simulink model "orion_casestudy_8"  (R2023a)
settings: Solver=VariableStepAuto  StartTime=0.0  StopTime=30  RelTol=1e-3
InitFcn:
  | RandStream.setGlobalStream(RandStream('mt19937ar','seed',sum(100*clock)));
undefined symbols (not defined in the file or in its folder): m, n
(part 1 of 3)
settings Model: Creator=simon  LastModifiedBy=simon
settings OptimizationCC: AccelVerboseBuild=on
settings DebuggingCC: UnderSpecifiedDataTypeMsg=warning  UnderSpecifiedDimensionMsg=warning

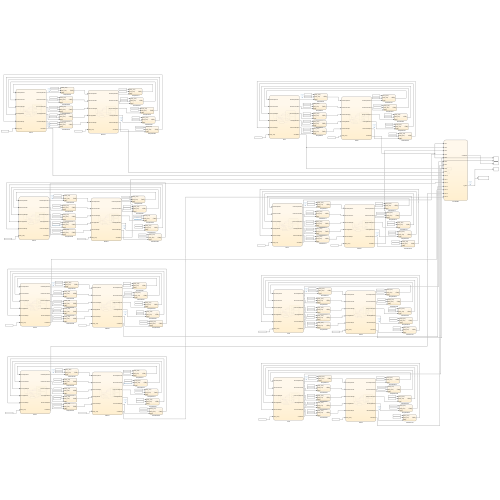
[thumbnail: Simulink's stored preview of the top-level diagram]
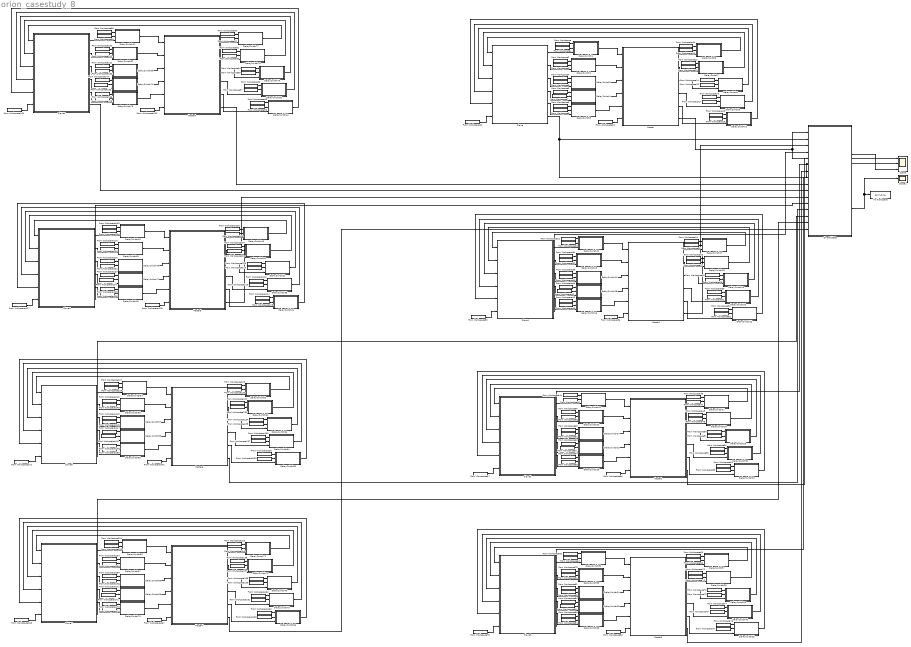
== system orion_casestudy_8 ==
  DelaySwitch1 : Stateflow chart  TreatAsAtomicUnit=on
  DelaySwitch10 : Stateflow chart  TreatAsAtomicUnit=on
  DelaySwitch11 : Stateflow chart  TreatAsAtomicUnit=on
  DelaySwitch12 : Stateflow chart  TreatAsAtomicUnit=on
  DelaySwitch13 : Stateflow chart  TreatAsAtomicUnit=on
  DelaySwitch14 : Stateflow chart  TreatAsAtomicUnit=on
  DelaySwitch15 : Stateflow chart  TreatAsAtomicUnit=on
  DelaySwitch16 : Stateflow chart  TreatAsAtomicUnit=on
  DelaySwitch17 : Stateflow chart  TreatAsAtomicUnit=on
  DelaySwitch18 : Stateflow chart  TreatAsAtomicUnit=on
  DelaySwitch19 : Stateflow chart  TreatAsAtomicUnit=on
  DelaySwitch2 : Stateflow chart  TreatAsAtomicUnit=on
  DelaySwitch20 : Stateflow chart  TreatAsAtomicUnit=on
  DelaySwitch21 : Stateflow chart  TreatAsAtomicUnit=on
  DelaySwitch22 : Stateflow chart  TreatAsAtomicUnit=on
  DelaySwitch23 : Stateflow chart  TreatAsAtomicUnit=on
  DelaySwitch24 : Stateflow chart  TreatAsAtomicUnit=on
  DelaySwitch25 : Stateflow chart  TreatAsAtomicUnit=on
  DelaySwitch26 : Stateflow chart  TreatAsAtomicUnit=on
  DelaySwitch27 : Stateflow chart  TreatAsAtomicUnit=on
  DelaySwitch28 : Stateflow chart  TreatAsAtomicUnit=on
  DelaySwitch29 : Stateflow chart  TreatAsAtomicUnit=on
  DelaySwitch3 : Stateflow chart  TreatAsAtomicUnit=on
  DelaySwitch30 : Stateflow chart  TreatAsAtomicUnit=on
  DelaySwitch31 : Stateflow chart  TreatAsAtomicUnit=on
  DelaySwitch32 : Stateflow chart  TreatAsAtomicUnit=on
  DelaySwitch33 : Stateflow chart  TreatAsAtomicUnit=on
  DelaySwitch34 : Stateflow chart  TreatAsAtomicUnit=on
  DelaySwitch35 : Stateflow chart  TreatAsAtomicUnit=on
  DelaySwitch36 : Stateflow chart  TreatAsAtomicUnit=on
  DelaySwitch37 : Stateflow chart  TreatAsAtomicUnit=on
  DelaySwitch38 : Stateflow chart  TreatAsAtomicUnit=on
  DelaySwitch39 : Stateflow chart  TreatAsAtomicUnit=on
  DelaySwitch4 : Stateflow chart  TreatAsAtomicUnit=on
  DelaySwitch40 : Stateflow chart  TreatAsAtomicUnit=on
  DelaySwitch41 : Stateflow chart  TreatAsAtomicUnit=on
  DelaySwitch42 : Stateflow chart  TreatAsAtomicUnit=on
  DelaySwitch43 : Stateflow chart  TreatAsAtomicUnit=on
  DelaySwitch44 : Stateflow chart  TreatAsAtomicUnit=on
  DelaySwitch45 : Stateflow chart  TreatAsAtomicUnit=on
  DelaySwitch46 : Stateflow chart  TreatAsAtomicUnit=on
  DelaySwitch47 : Stateflow chart  TreatAsAtomicUnit=on
  DelaySwitch48 : Stateflow chart  TreatAsAtomicUnit=on
  DelaySwitch49 : Stateflow chart  TreatAsAtomicUnit=on
  DelaySwitch5 : Stateflow chart  TreatAsAtomicUnit=on
  DelaySwitch50 : Stateflow chart  TreatAsAtomicUnit=on
  DelaySwitch51 : Stateflow chart  TreatAsAtomicUnit=on
  DelaySwitch52 : Stateflow chart  TreatAsAtomicUnit=on
  DelaySwitch53 : Stateflow chart  TreatAsAtomicUnit=on
  DelaySwitch54 : Stateflow chart  TreatAsAtomicUnit=on
  DelaySwitch55 : Stateflow chart  TreatAsAtomicUnit=on
  DelaySwitch56 : Stateflow chart  TreatAsAtomicUnit=on
  DelaySwitch57 : Stateflow chart  TreatAsAtomicUnit=on
  DelaySwitch58 : Stateflow chart  TreatAsAtomicUnit=on
  DelaySwitch59 : Stateflow chart  TreatAsAtomicUnit=on
  DelaySwitch6 : Stateflow chart  TreatAsAtomicUnit=on
  DelaySwitch60 : Stateflow chart  TreatAsAtomicUnit=on
  DelaySwitch61 : Stateflow chart  TreatAsAtomicUnit=on
  DelaySwitch62 : Stateflow chart  TreatAsAtomicUnit=on
  DelaySwitch63 : Stateflow chart  TreatAsAtomicUnit=on
  DelaySwitch64 : Stateflow chart  TreatAsAtomicUnit=on
  DelaySwitch65 : Stateflow chart  TreatAsAtomicUnit=on
  DelaySwitch66 : Stateflow chart  TreatAsAtomicUnit=on
  DelaySwitch67 : Stateflow chart  TreatAsAtomicUnit=on
  DelaySwitch68 : Stateflow chart  TreatAsAtomicUnit=on
  DelaySwitch69 : Stateflow chart  TreatAsAtomicUnit=on
  DelaySwitch7 : Stateflow chart  TreatAsAtomicUnit=on
  DelaySwitch70 : Stateflow chart  TreatAsAtomicUnit=on
  DelaySwitch71 : Stateflow chart  TreatAsAtomicUnit=on
  DelaySwitch72 : Stateflow chart  TreatAsAtomicUnit=on
  DelaySwitch73 : Stateflow chart  TreatAsAtomicUnit=on
  DelaySwitch74 : Stateflow chart  TreatAsAtomicUnit=on
  DelaySwitch75 : Stateflow chart  TreatAsAtomicUnit=on
  DelaySwitch76 : Stateflow chart  TreatAsAtomicUnit=on
  DelaySwitch77 : Stateflow chart  TreatAsAtomicUnit=on
  DelaySwitch78 : Stateflow chart  TreatAsAtomicUnit=on
  DelaySwitch79 : Stateflow chart  TreatAsAtomicUnit=on
  DelaySwitch8 : Stateflow chart  TreatAsAtomicUnit=on
  DelaySwitch80 : Stateflow chart  TreatAsAtomicUnit=on
  DelaySwitch9 : Stateflow chart  TreatAsAtomicUnit=on
  From Workspace : FromWorkspace  VariableName=switch_array_1  SampleTime=-1  Interpolate=off  ZeroCross=off  OutputAfterFinalValue=Holding final value
  From Workspace1 : FromWorkspace  VariableName=delay_array_1  SampleTime=-1  Interpolate=off  ZeroCross=off  OutputAfterFinalValue=Holding final value
  From Workspace10 : FromWorkspace  VariableName=switch_array_6  SampleTime=-1  Interpolate=off  ZeroCross=off  OutputAfterFinalValue=Holding final value
  From Workspace100 : FromWorkspace  VariableName=switch_array_52  SampleTime=-1  Interpolate=off  ZeroCross=off  OutputAfterFinalValue=Holding final value
  From Workspace101 : FromWorkspace  VariableName=delay_array_S5  SampleTime=-1  Interpolate=off  ZeroCross=off  OutputAfterFinalValue=Holding final value
  From Workspace102 : FromWorkspace  VariableName=delay_array_M5  SampleTime=-1  Interpolate=off  ZeroCross=off  OutputAfterFinalValue=Holding final value
  From Workspace103 : FromWorkspace  VariableName=switch_array_61  SampleTime=-1  Interpolate=off  ZeroCross=off  OutputAfterFinalValue=Holding final value
  From Workspace104 : FromWorkspace  VariableName=delay_array_61  SampleTime=-1  Interpolate=off  ZeroCross=off  OutputAfterFinalValue=Holding final value
  From Workspace105 : FromWorkspace  VariableName=switch_array_66  SampleTime=-1  Interpolate=off  ZeroCross=off  OutputAfterFinalValue=Holding final value
  From Workspace106 : FromWorkspace  VariableName=delay_array_66  SampleTime=-1  Interpolate=off  ZeroCross=off  OutputAfterFinalValue=Holding final value
  From Workspace107 : FromWorkspace  VariableName=switch_array_67  SampleTime=-1  Interpolate=off  ZeroCross=off  OutputAfterFinalValue=Holding final value
  From Workspace108 : FromWorkspace  VariableName=delay_array_67  SampleTime=-1  Interpolate=off  ZeroCross=off  OutputAfterFinalValue=Holding final value
  From Workspace109 : FromWorkspace  VariableName=switch_array_68  SampleTime=-1  Interpolate=off  ZeroCross=off  OutputAfterFinalValue=Holding final value
  From Workspace11 : FromWorkspace  VariableName=delay_array_6  SampleTime=-1  Interpolate=off  ZeroCross=off  OutputAfterFinalValue=Holding final value
  From Workspace110 : FromWorkspace  VariableName=delay_array_68  SampleTime=-1  Interpolate=off  ZeroCross=off  OutputAfterFinalValue=Holding final value
  From Workspace111 : FromWorkspace  VariableName=delay_array_52  SampleTime=-1  Interpolate=off  ZeroCross=off  OutputAfterFinalValue=Holding final value
  From Workspace112 : FromWorkspace  VariableName=switch_array_69  SampleTime=-1  Interpolate=off  ZeroCross=off  OutputAfterFinalValue=Holding final value
  From Workspace113 : FromWorkspace  VariableName=delay_array_69  SampleTime=-1  Interpolate=off  ZeroCross=off  OutputAfterFinalValue=Holding final value
  From Workspace114 : FromWorkspace  VariableName=switch_array_70  SampleTime=-1  Interpolate=off  ZeroCross=off  OutputAfterFinalValue=Holding final value
  From Workspace115 : FromWorkspace  VariableName=delay_array_70  SampleTime=-1  Interpolate=off  ZeroCross=off  OutputAfterFinalValue=Holding final value
  From Workspace116 : FromWorkspace  VariableName=switch_array_62  SampleTime=-1  Interpolate=off  ZeroCross=off  OutputAfterFinalValue=Holding final value
  From Workspace117 : FromWorkspace  VariableName=delay_array_S6  SampleTime=-1  Interpolate=off  ZeroCross=off  OutputAfterFinalValue=Holding final value
  From Workspace118 : FromWorkspace  VariableName=delay_array_M6  SampleTime=-1  Interpolate=off  ZeroCross=off  OutputAfterFinalValue=Holding final value
  From Workspace119 : FromWorkspace  VariableName=delay_array_62  SampleTime=-1  Interpolate=off  ZeroCross=off  OutputAfterFinalValue=Holding final value
  From Workspace12 : FromWorkspace  VariableName=switch_array_7  SampleTime=-1  Interpolate=off  ZeroCross=off  OutputAfterFinalValue=Holding final value
  From Workspace120 : FromWorkspace  VariableName=switch_array_63  SampleTime=-1  Interpolate=off  ZeroCross=off  OutputAfterFinalValue=Holding final value
  From Workspace121 : FromWorkspace  VariableName=delay_array_63  SampleTime=-1  Interpolate=off  ZeroCross=off  OutputAfterFinalValue=Holding final value
  From Workspace122 : FromWorkspace  VariableName=switch_array_53  SampleTime=-1  Interpolate=off  ZeroCross=off  OutputAfterFinalValue=Holding final value
  From Workspace123 : FromWorkspace  VariableName=switch_array_64  SampleTime=-1  Interpolate=off  ZeroCross=off  OutputAfterFinalValue=Holding final value
  From Workspace124 : FromWorkspace  VariableName=delay_array_64  SampleTime=-1  Interpolate=off  ZeroCross=off  OutputAfterFinalValue=Holding final value
  From Workspace125 : FromWorkspace  VariableName=switch_array_65  SampleTime=-1  Interpolate=off  ZeroCross=off  OutputAfterFinalValue=Holding final value
  From Workspace126 : FromWorkspace  VariableName=delay_array_65  SampleTime=-1  Interpolate=off  ZeroCross=off  OutputAfterFinalValue=Holding final value
  From Workspace127 : FromWorkspace  VariableName=switch_array_71  SampleTime=-1  Interpolate=off  ZeroCross=off  OutputAfterFinalValue=Holding final value
  From Workspace128 : FromWorkspace  VariableName=delay_array_71  SampleTime=-1  Interpolate=off  ZeroCross=off  OutputAfterFinalValue=Holding final value
  From Workspace129 : FromWorkspace  VariableName=switch_array_76  SampleTime=-1  Interpolate=off  ZeroCross=off  OutputAfterFinalValue=Holding final value
  From Workspace13 : FromWorkspace  VariableName=delay_array_7  SampleTime=-1  Interpolate=off  ZeroCross=off  OutputAfterFinalValue=Holding final value
  From Workspace130 : FromWorkspace  VariableName=delay_array_76  SampleTime=-1  Interpolate=off  ZeroCross=off  OutputAfterFinalValue=Holding final value
  From Workspace131 : FromWorkspace  VariableName=switch_array_77  SampleTime=-1  Interpolate=off  ZeroCross=off  OutputAfterFinalValue=Holding final value
  From Workspace132 : FromWorkspace  VariableName=delay_array_77  SampleTime=-1  Interpolate=off  ZeroCross=off  OutputAfterFinalValue=Holding final value
  From Workspace133 : FromWorkspace  VariableName=delay_array_53  SampleTime=-1  Interpolate=off  ZeroCross=off  OutputAfterFinalValue=Holding final value
  From Workspace134 : FromWorkspace  VariableName=switch_array_78  SampleTime=-1  Interpolate=off  ZeroCross=off  OutputAfterFinalValue=Holding final value
  From Workspace135 : FromWorkspace  VariableName=delay_array_78  SampleTime=-1  Interpolate=off  ZeroCross=off  OutputAfterFinalValue=Holding final value
  From Workspace136 : FromWorkspace  VariableName=switch_array_79  SampleTime=-1  Interpolate=off  ZeroCross=off  OutputAfterFinalValue=Holding final value
  From Workspace137 : FromWorkspace  VariableName=delay_array_79  SampleTime=-1  Interpolate=off  ZeroCross=off  OutputAfterFinalValue=Holding final value
  From Workspace138 : FromWorkspace  VariableName=switch_array_80  SampleTime=-1  Interpolate=off  ZeroCross=off  OutputAfterFinalValue=Holding final value
  From Workspace139 : FromWorkspace  VariableName=delay_array_80  SampleTime=-1  Interpolate=off  ZeroCross=off  OutputAfterFinalValue=Holding final value
  From Workspace14 : FromWorkspace  VariableName=switch_array_8  SampleTime=-1  Interpolate=off  ZeroCross=off  OutputAfterFinalValue=Holding final value
  From Workspace140 : FromWorkspace  VariableName=switch_array_72  SampleTime=-1  Interpolate=off  ZeroCross=off  OutputAfterFinalValue=Holding final value
  From Workspace141 : FromWorkspace  VariableName=delay_array_S7  SampleTime=-1  Interpolate=off  ZeroCross=off  OutputAfterFinalValue=Holding final value
  From Workspace142 : FromWorkspace  VariableName=delay_array_M7  SampleTime=-1  Interpolate=off  ZeroCross=off  OutputAfterFinalValue=Holding final value
  From Workspace143 : FromWorkspace  VariableName=delay_array_72  SampleTime=-1  Interpolate=off  ZeroCross=off  OutputAfterFinalValue=Holding final value
  From Workspace144 : FromWorkspace  VariableName=switch_array_54  SampleTime=-1  Interpolate=off  ZeroCross=off  OutputAfterFinalValue=Holding final value
  From Workspace145 : FromWorkspace  VariableName=switch_array_73  SampleTime=-1  Interpolate=off  ZeroCross=off  OutputAfterFinalValue=Holding final value
  From Workspace146 : FromWorkspace  VariableName=delay_array_73  SampleTime=-1  Interpolate=off  ZeroCross=off  OutputAfterFinalValue=Holding final value
  From Workspace147 : FromWorkspace  VariableName=switch_array_74  SampleTime=-1  Interpolate=off  ZeroCross=off  OutputAfterFinalValue=Holding final value
  From Workspace148 : FromWorkspace  VariableName=delay_array_74  SampleTime=-1  Interpolate=off  ZeroCross=off  OutputAfterFinalValue=Holding final value
  From Workspace149 : FromWorkspace  VariableName=switch_array_75  SampleTime=-1  Interpolate=off  ZeroCross=off  OutputAfterFinalValue=Holding final value
  From Workspace15 : FromWorkspace  VariableName=delay_array_8  SampleTime=-1  Interpolate=off  ZeroCross=off  OutputAfterFinalValue=Holding final value
  From Workspace150 : FromWorkspace  VariableName=delay_array_75  SampleTime=-1  Interpolate=off  ZeroCross=off  OutputAfterFinalValue=Holding final value
  From Workspace151 : FromWorkspace  VariableName=switch_array_81  SampleTime=-1  Interpolate=off  ZeroCross=off  OutputAfterFinalValue=Holding final value
  From Workspace152 : FromWorkspace  VariableName=delay_array_81  SampleTime=-1  Interpolate=off  ZeroCross=off  OutputAfterFinalValue=Holding final value
  From Workspace153 : FromWorkspace  VariableName=switch_array_86  SampleTime=-1  Interpolate=off  ZeroCross=off  OutputAfterFinalValue=Holding final value
  From Workspace154 : FromWorkspace  VariableName=delay_array_86  SampleTime=-1  Interpolate=off  ZeroCross=off  OutputAfterFinalValue=Holding final value
  From Workspace155 : FromWorkspace  VariableName=delay_array_54  SampleTime=-1  Interpolate=off  ZeroCross=off  OutputAfterFinalValue=Holding final value
  From Workspace156 : FromWorkspace  VariableName=switch_array_87  SampleTime=-1  Interpolate=off  ZeroCross=off  OutputAfterFinalValue=Holding final value
  From Workspace157 : FromWorkspace  VariableName=delay_array_87  SampleTime=-1  Interpolate=off  ZeroCross=off  OutputAfterFinalValue=Holding final value
  From Workspace158 : FromWorkspace  VariableName=switch_array_88  SampleTime=-1  Interpolate=off  ZeroCross=off  OutputAfterFinalValue=Holding final value
  From Workspace159 : FromWorkspace  VariableName=delay_array_88  SampleTime=-1  Interpolate=off  ZeroCross=off  OutputAfterFinalValue=Holding final value
  From Workspace16 : FromWorkspace  VariableName=switch_array_9  SampleTime=-1  Interpolate=off  ZeroCross=off  OutputAfterFinalValue=Holding final value
  From Workspace160 : FromWorkspace  VariableName=switch_array_89  SampleTime=-1  Interpolate=off  ZeroCross=off  OutputAfterFinalValue=Holding final value
  From Workspace161 : FromWorkspace  VariableName=delay_array_89  SampleTime=-1  Interpolate=off  ZeroCross=off  OutputAfterFinalValue=Holding final value
  From Workspace162 : FromWorkspace  VariableName=switch_array_90  SampleTime=-1  Interpolate=off  ZeroCross=off  OutputAfterFinalValue=Holding final value
  From Workspace163 : FromWorkspace  VariableName=delay_array_90  SampleTime=-1  Interpolate=off  ZeroCross=off  OutputAfterFinalValue=Holding final value
  From Workspace164 : FromWorkspace  VariableName=switch_array_82  SampleTime=-1  Interpolate=off  ZeroCross=off  OutputAfterFinalValue=Holding final value
  From Workspace165 : FromWorkspace  VariableName=delay_array_S8  SampleTime=-1  Interpolate=off  ZeroCross=off  OutputAfterFinalValue=Holding final value
  From Workspace166 : FromWorkspace  VariableName=switch_array_55  SampleTime=-1  Interpolate=off  ZeroCross=off  OutputAfterFinalValue=Holding final value
  From Workspace167 : FromWorkspace  VariableName=delay_array_M8  SampleTime=-1  Interpolate=off  ZeroCross=off  OutputAfterFinalValue=Holding final value
  From Workspace168 : FromWorkspace  VariableName=delay_array_82  SampleTime=-1  Interpolate=off  ZeroCross=off  OutputAfterFinalValue=Holding final value
  From Workspace169 : FromWorkspace  VariableName=switch_array_83  SampleTime=-1  Interpolate=off  ZeroCross=off  OutputAfterFinalValue=Holding final value
  From Workspace17 : FromWorkspace  VariableName=delay_array_9  SampleTime=-1  Interpolate=off  ZeroCross=off  OutputAfterFinalValue=Holding final value
  From Workspace170 : FromWorkspace  VariableName=delay_array_83  SampleTime=-1  Interpolate=off  ZeroCross=off  OutputAfterFinalValue=Holding final value
  From Workspace171 : FromWorkspace  VariableName=switch_array_84  SampleTime=-1  Interpolate=off  ZeroCross=off  OutputAfterFinalValue=Holding final value
  From Workspace172 : FromWorkspace  VariableName=delay_array_84  SampleTime=-1  Interpolate=off  ZeroCross=off  OutputAfterFinalValue=Holding final value
  From Workspace173 : FromWorkspace  VariableName=switch_array_85  SampleTime=-1  Interpolate=off  ZeroCross=off  OutputAfterFinalValue=Holding final value
  From Workspace174 : FromWorkspace  VariableName=delay_array_85  SampleTime=-1  Interpolate=off  ZeroCross=off  OutputAfterFinalValue=Holding final value
  From Workspace175 : FromWorkspace  VariableName=delay_array_55  SampleTime=-1  Interpolate=off  ZeroCross=off  OutputAfterFinalValue=Holding final value
  From Workspace18 : FromWorkspace  VariableName=switch_array_10  SampleTime=-1  Interpolate=off  ZeroCross=off  OutputAfterFinalValue=Holding final value
  From Workspace19 : FromWorkspace  VariableName=delay_array_10  SampleTime=-1  Interpolate=off  ZeroCross=off  OutputAfterFinalValue=Holding final value
  From Workspace2 : FromWorkspace  VariableName=switch_array_2  SampleTime=-1  Interpolate=off  ZeroCross=off  OutputAfterFinalValue=Holding final value
  From Workspace20 : FromWorkspace  VariableName=delay_array_S1  SampleTime=-1  Interpolate=off  ZeroCross=off  OutputAfterFinalValue=Holding final value
  From Workspace21 : FromWorkspace  VariableName=delay_array_M1  SampleTime=-1  Interpolate=off  ZeroCross=off  OutputAfterFinalValue=Holding final value
  From Workspace22 : FromWorkspace  VariableName=switch_array_11  SampleTime=-1  Interpolate=off  ZeroCross=off  OutputAfterFinalValue=Holding final value
  From Workspace23 : FromWorkspace  VariableName=delay_array_11  SampleTime=-1  Interpolate=off  ZeroCross=off  OutputAfterFinalValue=Holding final value
  From Workspace24 : FromWorkspace  VariableName=switch_array_16  SampleTime=-1  Interpolate=off  ZeroCross=off  OutputAfterFinalValue=Holding final value
  From Workspace25 : FromWorkspace  VariableName=delay_array_16  SampleTime=-1  Interpolate=off  ZeroCross=off  OutputAfterFinalValue=Holding final value
  From Workspace26 : FromWorkspace  VariableName=switch_array_17  SampleTime=-1  Interpolate=off  ZeroCross=off  OutputAfterFinalValue=Holding final value
  From Workspace27 : FromWorkspace  VariableName=delay_array_17  SampleTime=-1  Interpolate=off  ZeroCross=off  OutputAfterFinalValue=Holding final value
  From Workspace28 : FromWorkspace  VariableName=switch_array_18  SampleTime=-1  Interpolate=off  ZeroCross=off  OutputAfterFinalValue=Holding final value
  From Workspace29 : FromWorkspace  VariableName=delay_array_18  SampleTime=-1  Interpolate=off  ZeroCross=off  OutputAfterFinalValue=Holding final value
  From Workspace3 : FromWorkspace  VariableName=delay_array_2  SampleTime=-1  Interpolate=off  ZeroCross=off  OutputAfterFinalValue=Holding final value
  From Workspace30 : FromWorkspace  VariableName=switch_array_19  SampleTime=-1  Interpolate=off  ZeroCross=off  OutputAfterFinalValue=Holding final value
  From Workspace31 : FromWorkspace  VariableName=delay_array_19  SampleTime=-1  Interpolate=off  ZeroCross=off  OutputAfterFinalValue=Holding final value
  From Workspace32 : FromWorkspace  VariableName=switch_array_20  SampleTime=-1  Interpolate=off  ZeroCross=off  OutputAfterFinalValue=Holding final value
  From Workspace33 : FromWorkspace  VariableName=delay_array_20  SampleTime=-1  Interpolate=off  ZeroCross=off  OutputAfterFinalValue=Holding final value
  From Workspace34 : FromWorkspace  VariableName=switch_array_12  SampleTime=-1  Interpolate=off  ZeroCross=off  OutputAfterFinalValue=Holding final value
  From Workspace35 : FromWorkspace  VariableName=delay_array_S2  SampleTime=-1  Interpolate=off  ZeroCross=off  OutputAfterFinalValue=Holding final value
  From Workspace36 : FromWorkspace  VariableName=delay_array_M2  SampleTime=-1  Interpolate=off  ZeroCross=off  OutputAfterFinalValue=Holding final value
  From Workspace37 : FromWorkspace  VariableName=delay_array_12  SampleTime=-1  Interpolate=off  ZeroCross=off  OutputAfterFinalValue=Holding final value
  From Workspace38 : FromWorkspace  VariableName=switch_array_13  SampleTime=-1  Interpolate=off  ZeroCross=off  OutputAfterFinalValue=Holding final value
  From Workspace39 : FromWorkspace  VariableName=delay_array_13  SampleTime=-1  Interpolate=off  ZeroCross=off  OutputAfterFinalValue=Holding final value
  From Workspace4 : FromWorkspace  VariableName=switch_array_3  SampleTime=-1  Interpolate=off  ZeroCross=off  OutputAfterFinalValue=Holding final value
  From Workspace40 : FromWorkspace  VariableName=switch_array_14  SampleTime=-1  Interpolate=off  ZeroCross=off  OutputAfterFinalValue=Holding final value
  From Workspace41 : FromWorkspace  VariableName=delay_array_14  SampleTime=-1  Interpolate=off  ZeroCross=off  OutputAfterFinalValue=Holding final value
  From Workspace42 : FromWorkspace  VariableName=switch_array_15  SampleTime=-1  Interpolate=off  ZeroCross=off  OutputAfterFinalValue=Holding final value
  From Workspace43 : FromWorkspace  VariableName=delay_array_15  SampleTime=-1  Interpolate=off  ZeroCross=off  OutputAfterFinalValue=Holding final value
  From Workspace44 : FromWorkspace  VariableName=switch_array_31  SampleTime=-1  Interpolate=off  ZeroCross=off  OutputAfterFinalValue=Holding final value
  From Workspace45 : FromWorkspace  VariableName=delay_array_31  SampleTime=-1  Interpolate=off  ZeroCross=off  OutputAfterFinalValue=Holding final value
  From Workspace46 : FromWorkspace  VariableName=switch_array_36  SampleTime=-1  Interpolate=off  ZeroCross=off  OutputAfterFinalValue=Holding final value
  From Workspace47 : FromWorkspace  VariableName=delay_array_36  SampleTime=-1  Interpolate=off  ZeroCross=off  OutputAfterFinalValue=Holding final value
  From Workspace48 : FromWorkspace  VariableName=switch_array_37  SampleTime=-1  Interpolate=off  ZeroCross=off  OutputAfterFinalValue=Holding final value
  From Workspace49 : FromWorkspace  VariableName=delay_array_37  SampleTime=-1  Interpolate=off  ZeroCross=off  OutputAfterFinalValue=Holding final value
  From Workspace5 : FromWorkspace  VariableName=delay_array_3  SampleTime=-1  Interpolate=off  ZeroCross=off  OutputAfterFinalValue=Holding final value
  From Workspace50 : FromWorkspace  VariableName=switch_array_38  SampleTime=-1  Interpolate=off  ZeroCross=off  OutputAfterFinalValue=Holding final value
  From Workspace51 : FromWorkspace  VariableName=delay_array_38  SampleTime=-1  Interpolate=off  ZeroCross=off  OutputAfterFinalValue=Holding final value
  From Workspace52 : FromWorkspace  VariableName=switch_array_39  SampleTime=-1  Interpolate=off  ZeroCross=off  OutputAfterFinalValue=Holding final value
  From Workspace53 : FromWorkspace  VariableName=delay_array_39  SampleTime=-1  Interpolate=off  ZeroCross=off  OutputAfterFinalValue=Holding final value
  From Workspace54 : FromWorkspace  VariableName=switch_array_40  SampleTime=-1  Interpolate=off  ZeroCross=off  OutputAfterFinalValue=Holding final value
  From Workspace55 : FromWorkspace  VariableName=delay_array_40  SampleTime=-1  Interpolate=off  ZeroCross=off  OutputAfterFinalValue=Holding final value
  From Workspace56 : FromWorkspace  VariableName=switch_array_32  SampleTime=-1  Interpolate=off  ZeroCross=off  OutputAfterFinalValue=Holding final value
  From Workspace57 : FromWorkspace  VariableName=delay_array_S3  SampleTime=-1  Interpolate=off  ZeroCross=off  OutputAfterFinalValue=Holding final value
  From Workspace58 : FromWorkspace  VariableName=delay_array_M3  SampleTime=-1  Interpolate=off  ZeroCross=off  OutputAfterFinalValue=Holding final value
  From Workspace59 : FromWorkspace  VariableName=delay_array_32  SampleTime=-1  Interpolate=off  ZeroCross=off  OutputAfterFinalValue=Holding final value
  From Workspace6 : FromWorkspace  VariableName=switch_array_4  SampleTime=-1  Interpolate=off  ZeroCross=off  OutputAfterFinalValue=Holding final value
  From Workspace60 : FromWorkspace  VariableName=switch_array_33  SampleTime=-1  Interpolate=off  ZeroCross=off  OutputAfterFinalValue=Holding final value
  From Workspace61 : FromWorkspace  VariableName=delay_array_33  SampleTime=-1  Interpolate=off  ZeroCross=off  OutputAfterFinalValue=Holding final value
  From Workspace62 : FromWorkspace  VariableName=switch_array_34  SampleTime=-1  Interpolate=off  ZeroCross=off  OutputAfterFinalValue=Holding final value
  From Workspace63 : FromWorkspace  VariableName=delay_array_34  SampleTime=-1  Interpolate=off  ZeroCross=off  OutputAfterFinalValue=Holding final value
  From Workspace64 : FromWorkspace  VariableName=switch_array_35  SampleTime=-1  Interpolate=off  ZeroCross=off  OutputAfterFinalValue=Holding final value
  From Workspace65 : FromWorkspace  VariableName=delay_array_35  SampleTime=-1  Interpolate=off  ZeroCross=off  OutputAfterFinalValue=Holding final value
  From Workspace66 : FromWorkspace  VariableName=switch_array_41  SampleTime=-1  Interpolate=off  ZeroCross=off  OutputAfterFinalValue=Holding final value
  From Workspace67 : FromWorkspace  VariableName=delay_array_41  SampleTime=-1  Interpolate=off  ZeroCross=off  OutputAfterFinalValue=Holding final value
  From Workspace68 : FromWorkspace  VariableName=switch_array_46  SampleTime=-1  Interpolate=off  ZeroCross=off  OutputAfterFinalValue=Holding final value
  From Workspace69 : FromWorkspace  VariableName=delay_array_46  SampleTime=-1  Interpolate=off  ZeroCross=off  OutputAfterFinalValue=Holding final value
  From Workspace7 : FromWorkspace  VariableName=delay_array_4  SampleTime=-1  Interpolate=off  ZeroCross=off  OutputAfterFinalValue=Holding final value
  From Workspace70 : FromWorkspace  VariableName=switch_array_47  SampleTime=-1  Interpolate=off  ZeroCross=off  OutputAfterFinalValue=Holding final value
  From Workspace71 : FromWorkspace  VariableName=delay_array_47  SampleTime=-1  Interpolate=off  ZeroCross=off  OutputAfterFinalValue=Holding final value
  From Workspace72 : FromWorkspace  VariableName=switch_array_48  SampleTime=-1  Interpolate=off  ZeroCross=off  OutputAfterFinalValue=Holding final value
  From Workspace73 : FromWorkspace  VariableName=delay_array_48  SampleTime=-1  Interpolate=off  ZeroCross=off  OutputAfterFinalValue=Holding final value
  From Workspace74 : FromWorkspace  VariableName=switch_array_49  SampleTime=-1  Interpolate=off  ZeroCross=off  OutputAfterFinalValue=Holding final value
  From Workspace75 : FromWorkspace  VariableName=delay_array_49  SampleTime=-1  Interpolate=off  ZeroCross=off  OutputAfterFinalValue=Holding final value
  From Workspace76 : FromWorkspace  VariableName=switch_array_50  SampleTime=-1  Interpolate=off  ZeroCross=off  OutputAfterFinalValue=Holding final value
  From Workspace77 : FromWorkspace  VariableName=delay_array_50  SampleTime=-1  Interpolate=off  ZeroCross=off  OutputAfterFinalValue=Holding final value
  From Workspace78 : FromWorkspace  VariableName=switch_array_42  SampleTime=-1  Interpolate=off  ZeroCross=off  OutputAfterFinalValue=Holding final value
  From Workspace79 : FromWorkspace  VariableName=delay_array_S4  SampleTime=-1  Interpolate=off  ZeroCross=off  OutputAfterFinalValue=Holding final value
  From Workspace8 : FromWorkspace  VariableName=switch_array_5  SampleTime=-1  Interpolate=off  ZeroCross=off  OutputAfterFinalValue=Holding final value
  From Workspace80 : FromWorkspace  VariableName=delay_array_M4  SampleTime=-1  Interpolate=off  ZeroCross=off  OutputAfterFinalValue=Holding final value
  From Workspace81 : FromWorkspace  VariableName=delay_array_42  SampleTime=-1  Interpolate=off  ZeroCross=off  OutputAfterFinalValue=Holding final value
  From Workspace82 : FromWorkspace  VariableName=switch_array_43  SampleTime=-1  Interpolate=off  ZeroCross=off  OutputAfterFinalValue=Holding final value
  From Workspace83 : FromWorkspace  VariableName=delay_array_43  SampleTime=-1  Interpolate=off  ZeroCross=off  OutputAfterFinalValue=Holding final value
  From Workspace84 : FromWorkspace  VariableName=switch_array_44  SampleTime=-1  Interpolate=off  ZeroCross=off  OutputAfterFinalValue=Holding final value
  From Workspace85 : FromWorkspace  VariableName=delay_array_44  SampleTime=-1  Interpolate=off  ZeroCross=off  OutputAfterFinalValue=Holding final value
  From Workspace86 : FromWorkspace  VariableName=switch_array_45  SampleTime=-1  Interpolate=off  ZeroCross=off  OutputAfterFinalValue=Holding final value
  From Workspace87 : FromWorkspace  VariableName=delay_array_45  SampleTime=-1  Interpolate=off  ZeroCross=off  OutputAfterFinalValue=Holding final value
  From Workspace88 : FromWorkspace  VariableName=switch_array_51  SampleTime=-1  Interpolate=off  ZeroCross=off  OutputAfterFinalValue=Holding final value
  From Workspace89 : FromWorkspace  VariableName=delay_array_51  SampleTime=-1  Interpolate=off  ZeroCross=off  OutputAfterFinalValue=Holding final value
  From Workspace9 : FromWorkspace  VariableName=delay_array_5  SampleTime=-1  Interpolate=off  ZeroCross=off  OutputAfterFinalValue=Holding final value
  From Workspace90 : FromWorkspace  VariableName=switch_array_56  SampleTime=-1  Interpolate=off  ZeroCross=off  OutputAfterFinalValue=Holding final value
  From Workspace91 : FromWorkspace  VariableName=delay_array_56  SampleTime=-1  Interpolate=off  ZeroCross=off  OutputAfterFinalValue=Holding final value
  From Workspace92 : FromWorkspace  VariableName=switch_array_57  SampleTime=-1  Interpolate=off  ZeroCross=off  OutputAfterFinalValue=Holding final value
  From Workspace93 : FromWorkspace  VariableName=delay_array_57  SampleTime=-1  Interpolate=off  ZeroCross=off  OutputAfterFinalValue=Holding final value
  From Workspace94 : FromWorkspace  VariableName=switch_array_58  SampleTime=-1  Interpolate=off  ZeroCross=off  OutputAfterFinalValue=Holding final value
  From Workspace95 : FromWorkspace  VariableName=delay_array_58  SampleTime=-1  Interpolate=off  ZeroCross=off  OutputAfterFinalValue=Holding final value
  From Workspace96 : FromWorkspace  VariableName=switch_array_59  SampleTime=-1  Interpolate=off  ZeroCross=off  OutputAfterFinalValue=Holding final value
  From Workspace97 : FromWorkspace  VariableName=delay_array_59  SampleTime=-1  Interpolate=off  ZeroCross=off  OutputAfterFinalValue=Holding final value
  From Workspace98 : FromWorkspace  VariableName=switch_array_60  SampleTime=-1  Interpolate=off  ZeroCross=off  OutputAfterFinalValue=Holding final value
  From Workspace99 : FromWorkspace  VariableName=delay_array_60  SampleTime=-1  Interpolate=off  ZeroCross=off  OutputAfterFinalValue=Holding final value
  Master : Stateflow chart  TreatAsAtomicUnit=on
      settings: PortSchema="{\"entries\":[{\"content\":{\"sides\":[{\"content\":{\"connectorIds\":[\"In2\",\"In3\",\"In5\",\"In4\",\"In6\",\"In1\"]},\"type\":\"ConnectorPlacement.EquallySpacedRectSide\",\"uuid\":\"93190a42-59cb-4d31-aa72-080cef5549db\"},{\"content\":{\"connectorIds\":[\"Out1\",\"Out2\",\"Out3\",\"Out4\",\"Out5\",\"Out6\"],\"side\":\"RIGHT\"},\"type\":\"ConnectorPlacement.EquallySpacedRectSide\",\"uuid\":\"4a04e977-42e8-4d3e-8e66-86884aeb71d4\"},{\"content\":{\"side\":\"TOP\"},\"type\":\"ConnectorPlacement.EquallySpacedRectSide\",\"uuid\":\"cb7bc3bf-3799-42a3-9f12-c8b4e7be85f7\"},{\"content\":{\"side\":\"BOTTOM\"},\"type\":\"ConnectorPlacement.EquallySpacedRectSide\",\"uuid\":\"934a78a5-af7b-46d0-ad43-c65a76addb63\"}]},\"type\":\"ConnectorPlacement.EquallySpacedConnector\",\"uuid\":\"bab253c4-7746-42e8-9b4d-6fa7ff1cc3b1\"}],\"packageUris\":[\"http://schema.mathworks.com/mf0/Connector/R2020b\"],\"version\":\"1.0\"}"
  Master1 : Stateflow chart  TreatAsAtomicUnit=on
      settings: PortSchema="{\"entries\":[{\"content\":{\"sides\":[{\"content\":{\"connectorIds\":[\"In2\",\"In3\",\"In5\",\"In4\",\"In6\",\"In1\"]},\"type\":\"ConnectorPlacement.EquallySpacedRectSide\",\"uuid\":\"93190a42-59cb-4d31-aa72-080cef5549db\"},{\"content\":{\"connectorIds\":[\"Out1\",\"Out2\",\"Out3\",\"Out4\",\"Out5\",\"Out6\"],\"side\":\"RIGHT\"},\"type\":\"ConnectorPlacement.EquallySpacedRectSide\",\"uuid\":\"4a04e977-42e8-4d3e-8e66-86884aeb71d4\"},{\"content\":{\"side\":\"TOP\"},\"type\":\"ConnectorPlacement.EquallySpacedRectSide\",\"uuid\":\"cb7bc3bf-3799-42a3-9f12-c8b4e7be85f7\"},{\"content\":{\"side\":\"BOTTOM\"},\"type\":\"ConnectorPlacement.EquallySpacedRectSide\",\"uuid\":\"934a78a5-af7b-46d0-ad43-c65a76addb63\"}]},\"type\":\"ConnectorPlacement.EquallySpacedConnector\",\"uuid\":\"bab253c4-7746-42e8-9b4d-6fa7ff1cc3b1\"}],\"packageUris\":[\"http://schema.mathworks.com/mf0/Connector/R2020b\"],\"version\":\"1.0\"}"
  Master2 : Stateflow chart  TreatAsAtomicUnit=on
      settings: PortSchema="{\"entries\":[{\"content\":{\"sides\":[{\"content\":{\"connectorIds\":[\"In2\",\"In3\",\"In5\",\"In4\",\"In6\",\"In1\"]},\"type\":\"ConnectorPlacement.EquallySpacedRectSide\",\"uuid\":\"93190a42-59cb-4d31-aa72-080cef5549db\"},{\"content\":{\"connectorIds\":[\"Out1\",\"Out2\",\"Out3\",\"Out4\",\"Out5\",\"Out6\"],\"side\":\"RIGHT\"},\"type\":\"ConnectorPlacement.EquallySpacedRectSide\",\"uuid\":\"4a04e977-42e8-4d3e-8e66-86884aeb71d4\"},{\"content\":{\"side\":\"TOP\"},\"type\":\"ConnectorPlacement.EquallySpacedRectSide\",\"uuid\":\"cb7bc3bf-3799-42a3-9f12-c8b4e7be85f7\"},{\"content\":{\"side\":\"BOTTOM\"},\"type\":\"ConnectorPlacement.EquallySpacedRectSide\",\"uuid\":\"934a78a5-af7b-46d0-ad43-c65a76addb63\"}]},\"type\":\"ConnectorPlacement.EquallySpacedConnector\",\"uuid\":\"bab253c4-7746-42e8-9b4d-6fa7ff1cc3b1\"}],\"packageUris\":[\"http://schema.mathworks.com/mf0/Connector/R2020b\"],\"version\":\"1.0\"}"
  Master3 : Stateflow chart  TreatAsAtomicUnit=on
      settings: PortSchema="{\"entries\":[{\"content\":{\"sides\":[{\"content\":{\"connectorIds\":[\"In2\",\"In3\",\"In5\",\"In4\",\"In6\",\"In1\"]},\"type\":\"ConnectorPlacement.EquallySpacedRectSide\",\"uuid\":\"93190a42-59cb-4d31-aa72-080cef5549db\"},{\"content\":{\"connectorIds\":[\"Out1\",\"Out2\",\"Out3\",\"Out4\",\"Out5\",\"Out6\"],\"side\":\"RIGHT\"},\"type\":\"ConnectorPlacement.EquallySpacedRectSide\",\"uuid\":\"4a04e977-42e8-4d3e-8e66-86884aeb71d4\"},{\"content\":{\"side\":\"TOP\"},\"type\":\"ConnectorPlacement.EquallySpacedRectSide\",\"uuid\":\"cb7bc3bf-3799-42a3-9f12-c8b4e7be85f7\"},{\"content\":{\"side\":\"BOTTOM\"},\"type\":\"ConnectorPlacement.EquallySpacedRectSide\",\"uuid\":\"934a78a5-af7b-46d0-ad43-c65a76addb63\"}]},\"type\":\"ConnectorPlacement.EquallySpacedConnector\",\"uuid\":\"bab253c4-7746-42e8-9b4d-6fa7ff1cc3b1\"}],\"packageUris\":[\"http://schema.mathworks.com/mf0/Connector/R2020b\"],\"version\":\"1.0\"}"
  Master4 : Stateflow chart  TreatAsAtomicUnit=on
      settings: PortSchema="{\"entries\":[{\"content\":{\"sides\":[{\"content\":{\"connectorIds\":[\"In2\",\"In3\",\"In5\",\"In4\",\"In6\",\"In1\"]},\"type\":\"ConnectorPlacement.EquallySpacedRectSide\",\"uuid\":\"93190a42-59cb-4d31-aa72-080cef5549db\"},{\"content\":{\"connectorIds\":[\"Out1\",\"Out2\",\"Out3\",\"Out4\",\"Out5\",\"Out6\"],\"side\":\"RIGHT\"},\"type\":\"ConnectorPlacement.EquallySpacedRectSide\",\"uuid\":\"4a04e977-42e8-4d3e-8e66-86884aeb71d4\"},{\"content\":{\"side\":\"TOP\"},\"type\":\"ConnectorPlacement.EquallySpacedRectSide\",\"uuid\":\"cb7bc3bf-3799-42a3-9f12-c8b4e7be85f7\"},{\"content\":{\"side\":\"BOTTOM\"},\"type\":\"ConnectorPlacement.EquallySpacedRectSide\",\"uuid\":\"934a78a5-af7b-46d0-ad43-c65a76addb63\"}]},\"type\":\"ConnectorPlacement.EquallySpacedConnector\",\"uuid\":\"bab253c4-7746-42e8-9b4d-6fa7ff1cc3b1\"}],\"packageUris\":[\"http://schema.mathworks.com/mf0/Connector/R2020b\"],\"version\":\"1.0\"}"
  Master5 : Stateflow chart  TreatAsAtomicUnit=on
      settings: PortSchema="{\"entries\":[{\"content\":{\"sides\":[{\"content\":{\"connectorIds\":[\"In2\",\"In3\",\"In5\",\"In4\",\"In6\",\"In1\"]},\"type\":\"ConnectorPlacement.EquallySpacedRectSide\",\"uuid\":\"93190a42-59cb-4d31-aa72-080cef5549db\"},{\"content\":{\"connectorIds\":[\"Out1\",\"Out2\",\"Out3\",\"Out4\",\"Out5\",\"Out6\"],\"side\":\"RIGHT\"},\"type\":\"ConnectorPlacement.EquallySpacedRectSide\",\"uuid\":\"4a04e977-42e8-4d3e-8e66-86884aeb71d4\"},{\"content\":{\"side\":\"TOP\"},\"type\":\"ConnectorPlacement.EquallySpacedRectSide\",\"uuid\":\"cb7bc3bf-3799-42a3-9f12-c8b4e7be85f7\"},{\"content\":{\"side\":\"BOTTOM\"},\"type\":\"ConnectorPlacement.EquallySpacedRectSide\",\"uuid\":\"934a78a5-af7b-46d0-ad43-c65a76addb63\"}]},\"type\":\"ConnectorPlacement.EquallySpacedConnector\",\"uuid\":\"bab253c4-7746-42e8-9b4d-6fa7ff1cc3b1\"}],\"packageUris\":[\"http://schema.mathworks.com/mf0/Connector/R2020b\"],\"version\":\"1.0\"}"
  Master6 : Stateflow chart  TreatAsAtomicUnit=on
      settings: PortSchema="{\"entries\":[{\"content\":{\"sides\":[{\"content\":{\"connectorIds\":[\"In2\",\"In3\",\"In5\",\"In4\",\"In6\",\"In1\"]},\"type\":\"ConnectorPlacement.EquallySpacedRectSide\",\"uuid\":\"93190a42-59cb-4d31-aa72-080cef5549db\"},{\"content\":{\"connectorIds\":[\"Out1\",\"Out2\",\"Out3\",\"Out4\",\"Out5\",\"Out6\"],\"side\":\"RIGHT\"},\"type\":\"ConnectorPlacement.EquallySpacedRectSide\",\"uuid\":\"4a04e977-42e8-4d3e-8e66-86884aeb71d4\"},{\"content\":{\"side\":\"TOP\"},\"type\":\"ConnectorPlacement.EquallySpacedRectSide\",\"uuid\":\"cb7bc3bf-3799-42a3-9f12-c8b4e7be85f7\"},{\"content\":{\"side\":\"BOTTOM\"},\"type\":\"ConnectorPlacement.EquallySpacedRectSide\",\"uuid\":\"934a78a5-af7b-46d0-ad43-c65a76addb63\"}]},\"type\":\"ConnectorPlacement.EquallySpacedConnector\",\"uuid\":\"bab253c4-7746-42e8-9b4d-6fa7ff1cc3b1\"}],\"packageUris\":[\"http://schema.mathworks.com/mf0/Connector/R2020b\"],\"version\":\"1.0\"}"
  Master7 : Stateflow chart  TreatAsAtomicUnit=on
      settings: PortSchema="{\"entries\":[{\"content\":{\"sides\":[{\"content\":{\"connectorIds\":[\"In2\",\"In3\",\"In5\",\"In4\",\"In6\",\"In1\"]},\"type\":\"ConnectorPlacement.EquallySpacedRectSide\",\"uuid\":\"93190a42-59cb-4d31-aa72-080cef5549db\"},{\"content\":{\"connectorIds\":[\"Out1\",\"Out2\",\"Out3\",\"Out4\",\"Out5\",\"Out6\"],\"side\":\"RIGHT\"},\"type\":\"ConnectorPlacement.EquallySpacedRectSide\",\"uuid\":\"4a04e977-42e8-4d3e-8e66-86884aeb71d4\"},{\"content\":{\"side\":\"TOP\"},\"type\":\"ConnectorPlacement.EquallySpacedRectSide\",\"uuid\":\"cb7bc3bf-3799-42a3-9f12-c8b4e7be85f7\"},{\"content\":{\"side\":\"BOTTOM\"},\"type\":\"ConnectorPlacement.EquallySpacedRectSide\",\"uuid\":\"934a78a5-af7b-46d0-ad43-c65a76addb63\"}]},\"type\":\"ConnectorPlacement.EquallySpacedConnector\",\"uuid\":\"bab253c4-7746-42e8-9b4d-6fa7ff1cc3b1\"}],\"packageUris\":[\"http://schema.mathworks.com/mf0/Connector/R2020b\"],\"version\":\"1.0\"}"
  OverallState : Stateflow chart  TreatAsAtomicUnit=on
  Scope : Scope  NumInputPorts=3
  Scope1 : Scope
  Slave : Stateflow chart  TreatAsAtomicUnit=on
      settings: PortSchema="{\"entries\":[{\"content\":{\"sides\":[{\"content\":{\"connectorIds\":[\"In1\",\"In5\",\"In3\",\"In2\",\"In4\",\"In6\"]},\"type\":\"ConnectorPlacement.EquallySpacedRectSide\",\"uuid\":\"93190a42-59cb-4d31-aa72-080cef5549db\"},{\"content\":{\"connectorIds\":[\"Out3\",\"Out1\",\"Out2\",\"Out4\",\"Out5\",\"Out6\"],\"side\":\"RIGHT\"},\"type\":\"ConnectorPlacement.EquallySpacedRectSide\",\"uuid\":\"4a04e977-42e8-4d3e-8e66-86884aeb71d4\"},{\"content\":{\"side\":\"TOP\"},\"type\":\"ConnectorPlacement.EquallySpacedRectSide\",\"uuid\":\"cb7bc3bf-3799-42a3-9f12-c8b4e7be85f7\"}]},\"type\":\"ConnectorPlacement.EquallySpacedConnector\",\"uuid\":\"bab253c4-7746-42e8-9b4d-6fa7ff1cc3b1\"}],\"packageUris\":[\"http://schema.mathworks.com/mf0/Connector/R2020b\"],\"version\":\"1.0\"}"
  Slave1 : Stateflow chart  TreatAsAtomicUnit=on
      settings: PortSchema="{\"entries\":[{\"content\":{\"sides\":[{\"content\":{\"connectorIds\":[\"In1\",\"In5\",\"In3\",\"In2\",\"In4\",\"In6\"]},\"type\":\"ConnectorPlacement.EquallySpacedRectSide\",\"uuid\":\"93190a42-59cb-4d31-aa72-080cef5549db\"},{\"content\":{\"connectorIds\":[\"Out3\",\"Out1\",\"Out2\",\"Out4\",\"Out5\",\"Out6\"],\"side\":\"RIGHT\"},\"type\":\"ConnectorPlacement.EquallySpacedRectSide\",\"uuid\":\"4a04e977-42e8-4d3e-8e66-86884aeb71d4\"},{\"content\":{\"side\":\"TOP\"},\"type\":\"ConnectorPlacement.EquallySpacedRectSide\",\"uuid\":\"cb7bc3bf-3799-42a3-9f12-c8b4e7be85f7\"}]},\"type\":\"ConnectorPlacement.EquallySpacedConnector\",\"uuid\":\"bab253c4-7746-42e8-9b4d-6fa7ff1cc3b1\"}],\"packageUris\":[\"http://schema.mathworks.com/mf0/Connector/R2020b\"],\"version\":\"1.0\"}"
  Slave2 : Stateflow chart  TreatAsAtomicUnit=on
      settings: PortSchema="{\"entries\":[{\"content\":{\"sides\":[{\"content\":{\"connectorIds\":[\"In1\",\"In5\",\"In3\",\"In2\",\"In4\",\"In6\"]},\"type\":\"ConnectorPlacement.EquallySpacedRectSide\",\"uuid\":\"93190a42-59cb-4d31-aa72-080cef5549db\"},{\"content\":{\"connectorIds\":[\"Out3\",\"Out1\",\"Out2\",\"Out4\",\"Out5\",\"Out6\"],\"side\":\"RIGHT\"},\"type\":\"ConnectorPlacement.EquallySpacedRectSide\",\"uuid\":\"4a04e977-42e8-4d3e-8e66-86884aeb71d4\"},{\"content\":{\"side\":\"TOP\"},\"type\":\"ConnectorPlacement.EquallySpacedRectSide\",\"uuid\":\"cb7bc3bf-3799-42a3-9f12-c8b4e7be85f7\"}]},\"type\":\"ConnectorPlacement.EquallySpacedConnector\",\"uuid\":\"bab253c4-7746-42e8-9b4d-6fa7ff1cc3b1\"}],\"packageUris\":[\"http://schema.mathworks.com/mf0/Connector/R2020b\"],\"version\":\"1.0\"}"
  Slave3 : Stateflow chart  TreatAsAtomicUnit=on
      settings: PortSchema="{\"entries\":[{\"content\":{\"sides\":[{\"content\":{\"connectorIds\":[\"In1\",\"In5\",\"In3\",\"In2\",\"In4\",\"In6\"]},\"type\":\"ConnectorPlacement.EquallySpacedRectSide\",\"uuid\":\"93190a42-59cb-4d31-aa72-080cef5549db\"},{\"content\":{\"connectorIds\":[\"Out3\",\"Out1\",\"Out2\",\"Out4\",\"Out5\",\"Out6\"],\"side\":\"RIGHT\"},\"type\":\"ConnectorPlacement.EquallySpacedRectSide\",\"uuid\":\"4a04e977-42e8-4d3e-8e66-86884aeb71d4\"},{\"content\":{\"side\":\"TOP\"},\"type\":\"ConnectorPlacement.EquallySpacedRectSide\",\"uuid\":\"cb7bc3bf-3799-42a3-9f12-c8b4e7be85f7\"}]},\"type\":\"ConnectorPlacement.EquallySpacedConnector\",\"uuid\":\"bab253c4-7746-42e8-9b4d-6fa7ff1cc3b1\"}],\"packageUris\":[\"http://schema.mathworks.com/mf0/Connector/R2020b\"],\"version\":\"1.0\"}"
  Slave4 : Stateflow chart  TreatAsAtomicUnit=on
      settings: PortSchema="{\"entries\":[{\"content\":{\"sides\":[{\"content\":{\"connectorIds\":[\"In1\",\"In5\",\"In3\",\"In2\",\"In4\",\"In6\"]},\"type\":\"ConnectorPlacement.EquallySpacedRectSide\",\"uuid\":\"93190a42-59cb-4d31-aa72-080cef5549db\"},{\"content\":{\"connectorIds\":[\"Out3\",\"Out1\",\"Out2\",\"Out4\",\"Out5\",\"Out6\"],\"side\":\"RIGHT\"},\"type\":\"ConnectorPlacement.EquallySpacedRectSide\",\"uuid\":\"4a04e977-42e8-4d3e-8e66-86884aeb71d4\"},{\"content\":{\"side\":\"TOP\"},\"type\":\"ConnectorPlacement.EquallySpacedRectSide\",\"uuid\":\"cb7bc3bf-3799-42a3-9f12-c8b4e7be85f7\"}]},\"type\":\"ConnectorPlacement.EquallySpacedConnector\",\"uuid\":\"bab253c4-7746-42e8-9b4d-6fa7ff1cc3b1\"}],\"packageUris\":[\"http://schema.mathworks.com/mf0/Connector/R2020b\"],\"version\":\"1.0\"}"
  Slave5 : Stateflow chart  TreatAsAtomicUnit=on
      settings: PortSchema="{\"entries\":[{\"content\":{\"sides\":[{\"content\":{\"connectorIds\":[\"In1\",\"In5\",\"In3\",\"In2\",\"In4\",\"In6\"]},\"type\":\"ConnectorPlacement.EquallySpacedRectSide\",\"uuid\":\"93190a42-59cb-4d31-aa72-080cef5549db\"},{\"content\":{\"connectorIds\":[\"Out3\",\"Out1\",\"Out2\",\"Out4\",\"Out5\",\"Out6\"],\"side\":\"RIGHT\"},\"type\":\"ConnectorPlacement.EquallySpacedRectSide\",\"uuid\":\"4a04e977-42e8-4d3e-8e66-86884aeb71d4\"},{\"content\":{\"side\":\"TOP\"},\"type\":\"ConnectorPlacement.EquallySpacedRectSide\",\"uuid\":\"cb7bc3bf-3799-42a3-9f12-c8b4e7be85f7\"}]},\"type\":\"ConnectorPlacement.EquallySpacedConnector\",\"uuid\":\"bab253c4-7746-42e8-9b4d-6fa7ff1cc3b1\"}],\"packageUris\":[\"http://schema.mathworks.com/mf0/Connector/R2020b\"],\"version\":\"1.0\"}"
  Slave6 : Stateflow chart  TreatAsAtomicUnit=on
      settings: PortSchema="{\"entries\":[{\"content\":{\"sides\":[{\"content\":{\"connectorIds\":[\"In1\",\"In5\",\"In3\",\"In2\",\"In4\",\"In6\"]},\"type\":\"ConnectorPlacement.EquallySpacedRectSide\",\"uuid\":\"93190a42-59cb-4d31-aa72-080cef5549db\"},{\"content\":{\"connectorIds\":[\"Out3\",\"Out1\",\"Out2\",\"Out4\",\"Out5\",\"Out6\"],\"side\":\"RIGHT\"},\"type\":\"ConnectorPlacement.EquallySpacedRectSide\",\"uuid\":\"4a04e977-42e8-4d3e-8e66-86884aeb71d4\"},{\"content\":{\"side\":\"TOP\"},\"type\":\"ConnectorPlacement.EquallySpacedRectSide\",\"uuid\":\"cb7bc3bf-3799-42a3-9f12-c8b4e7be85f7\"}]},\"type\":\"ConnectorPlacement.EquallySpacedConnector\",\"uuid\":\"bab253c4-7746-42e8-9b4d-6fa7ff1cc3b1\"}],\"packageUris\":[\"http://schema.mathworks.com/mf0/Connector/R2020b\"],\"version\":\"1.0\"}"
  Slave7 : Stateflow chart  TreatAsAtomicUnit=on
      settings: PortSchema="{\"entries\":[{\"content\":{\"sides\":[{\"content\":{\"connectorIds\":[\"In1\",\"In5\",\"In3\",\"In2\",\"In4\",\"In6\"]},\"type\":\"ConnectorPlacement.EquallySpacedRectSide\",\"uuid\":\"93190a42-59cb-4d31-aa72-080cef5549db\"},{\"content\":{\"connectorIds\":[\"Out3\",\"Out1\",\"Out2\",\"Out4\",\"Out5\",\"Out6\"],\"side\":\"RIGHT\"},\"type\":\"ConnectorPlacement.EquallySpacedRectSide\",\"uuid\":\"4a04e977-42e8-4d3e-8e66-86884aeb71d4\"},{\"content\":{\"side\":\"TOP\"},\"type\":\"ConnectorPlacement.EquallySpacedRectSide\",\"uuid\":\"cb7bc3bf-3799-42a3-9f12-c8b4e7be85f7\"}]},\"type\":\"ConnectorPlacement.EquallySpacedConnector\",\"uuid\":\"bab253c4-7746-42e8-9b4d-6fa7ff1cc3b1\"}],\"packageUris\":[\"http://schema.mathworks.com/mf0/Connector/R2020b\"],\"version\":\"1.0\"}"
  To Workspace : ToWorkspace  VariableName=conn_time  SaveFormat=Timeseries  SampleTime=-1
  wires:
  Slave/4(OrionAppDataOut) -> DelaySwitch4/3(inMsg)
  Slave/2(OrionConnRespOut) -> DelaySwitch3/3(inMsg)
  Slave/1(OrionConnConfOut) -> DelaySwitch2/3(inMsg)
  Slave/3(OrionKeepAliveOut) -> DelaySwitch1/3(inMsg)
  DelaySwitch3/1(outMsg) -> Master/5(OrionConnRespIn)
  DelaySwitch4/1(outMsg) -> Master/4(OrionAppDataIn)
  DelaySwitch2/1(outMsg) -> Master/3(OrionConnConfIn)
  DelaySwitch1/1(outMsg) -> Master/2(OrionKeepAliveIn)
  DelaySwitch10/1(outMsg) -> Slave/4(OrionConnReqIn)
  DelaySwitch9/1(outMsg) -> Slave/2(OrionAppDataIn)
  DelaySwitch8/1(outMsg) -> Slave/3(OrionConnRespIn)
  DelaySwitch7/1(outMsg) -> Slave/5(OrionConnConfIn)
  DelaySwitch6/1(outMsg) -> Slave/1(OrionKeepAliveIn)
  Master/6(connStatus) -> Scope/1, OverallState/1(conn1)
  Slave/6(connStatus) -> Scope/2, OverallState/2(conn2)
  OverallState/1(connStatus) -> Scope/3
  OverallState/2(op_time) -> Scope1/1, To Workspace/1
  From Workspace/1 -> DelaySwitch1/1(switch_array)
  From Workspace1/1 -> DelaySwitch1/2(delay_array)
  From Workspace3/1 -> DelaySwitch2/2(delay_array)
  From Workspace2/1 -> DelaySwitch2/1(switch_array)
  From Workspace4/1 -> DelaySwitch3/1(switch_array)
  From Workspace5/1 -> DelaySwitch3/2(delay_array)
  From Workspace7/1 -> DelaySwitch4/2(delay_array)
  From Workspace6/1 -> DelaySwitch4/1(switch_array)
  From Workspace8/1 -> DelaySwitch5/1(switch_array)
  From Workspace9/1 -> DelaySwitch5/2(delay_array)
  Slave/5(OrionConnReqOut) -> DelaySwitch5/3(inMsg)
  DelaySwitch5/1(outMsg) -> Master/6(OrionConnReqIn)
  From Workspace11/1 -> DelaySwitch6/2(delay_array)
  From Workspace10/1 -> DelaySwitch6/1(switch_array)
  Master/1(OrionKeepAliveOut) -> DelaySwitch6/3(inMsg)
  From Workspace12/1 -> DelaySwitch7/1(switch_array)
  From Workspace13/1 -> DelaySwitch7/2(delay_array)
  From Workspace15/1 -> DelaySwitch8/2(delay_array)
  From Workspace14/1 -> DelaySwitch8/1(switch_array)
  Master/2(OrionConnConfOut) -> DelaySwitch7/3(inMsg)
  Master/3(OrionConnRespOut) -> DelaySwitch8/3(inMsg)
  From Workspace16/1 -> DelaySwitch9/1(switch_array)
  From Workspace17/1 -> DelaySwitch9/2(delay_array)
  From Workspace19/1 -> DelaySwitch10/2(delay_array)
  From Workspace18/1 -> DelaySwitch10/1(switch_array)
  Master/4(OrionAppDataOut) -> DelaySwitch9/3(inMsg)
  Master/5(OrionConnReqOut) -> DelaySwitch10/3(inMsg)
  From Workspace20/1 -> Slave/6(delay_array)
  From Workspace21/1 -> Master/1(delay_array)
  From Workspace36/1 -> Master1/1(delay_array)
  From Workspace35/1 -> Slave1/6(delay_array)
  Master1/5(OrionConnReqOut) -> DelaySwitch12/3(inMsg)
  Master1/4(OrionAppDataOut) -> DelaySwitch20/3(inMsg)
  From Workspace32/1 -> DelaySwitch12/1(switch_array)
  From Workspace33/1 -> DelaySwitch12/2(delay_array)
  From Workspace31/1 -> DelaySwitch20/2(delay_array)
  From Workspace30/1 -> DelaySwitch20/1(switch_array)
  Master1/3(OrionConnRespOut) -> DelaySwitch19/3(inMsg)
  Master1/2(OrionConnConfOut) -> DelaySwitch18/3(inMsg)
  From Workspace28/1 -> DelaySwitch19/1(switch_array)
  From Workspace29/1 -> DelaySwitch19/2(delay_array)
  From Workspace27/1 -> DelaySwitch18/2(delay_array)
  From Workspace26/1 -> DelaySwitch18/1(switch_array)
  Master1/1(OrionKeepAliveOut) -> DelaySwitch17/3(inMsg)
  From Workspace24/1 -> DelaySwitch17/1(switch_array)
  From Workspace25/1 -> DelaySwitch17/2(delay_array)
  DelaySwitch16/1(outMsg) -> Master1/6(OrionConnReqIn)
  Slave1/5(OrionConnReqOut) -> DelaySwitch16/3(inMsg)
  From Workspace43/1 -> DelaySwitch16/2(delay_array)
  From Workspace42/1 -> DelaySwitch16/1(switch_array)
  From Workspace40/1 -> DelaySwitch15/1(switch_array)
  From Workspace41/1 -> DelaySwitch15/2(delay_array)
  From Workspace39/1 -> DelaySwitch14/2(delay_array)
  From Workspace38/1 -> DelaySwitch14/1(switch_array)
  From Workspace34/1 -> DelaySwitch13/1(switch_array)
  From Workspace37/1 -> DelaySwitch13/2(delay_array)
  From Workspace23/1 -> DelaySwitch11/2(delay_array)
  From Workspace22/1 -> DelaySwitch11/1(switch_array)
  Slave1/6(connStatus) -> OverallState/4(conn4)
  Master1/6(connStatus) -> OverallState/3(conn3)
  DelaySwitch17/1(outMsg) -> Slave1/1(OrionKeepAliveIn)
  DelaySwitch18/1(outMsg) -> Slave1/5(OrionConnConfIn)
  DelaySwitch19/1(outMsg) -> Slave1/3(OrionConnRespIn)
  DelaySwitch20/1(outMsg) -> Slave1/2(OrionAppDataIn)
  DelaySwitch12/1(outMsg) -> Slave1/4(OrionConnReqIn)
  DelaySwitch11/1(outMsg) -> Master1/2(OrionKeepAliveIn)
  DelaySwitch13/1(outMsg) -> Master1/3(OrionConnConfIn)
  DelaySwitch15/1(outMsg) -> Master1/4(OrionAppDataIn)
  DelaySwitch14/1(outMsg) -> Master1/5(OrionConnRespIn)
  Slave1/3(OrionKeepAliveOut) -> DelaySwitch11/3(inMsg)
  Slave1/1(OrionConnConfOut) -> DelaySwitch13/3(inMsg)
  Slave1/2(OrionConnRespOut) -> DelaySwitch14/3(inMsg)
  Slave1/4(OrionAppDataOut) -> DelaySwitch15/3(inMsg)
  Slave2/4(OrionAppDataOut) -> DelaySwitch25/3(inMsg)
  Slave2/2(OrionConnRespOut) -> DelaySwitch24/3(inMsg)
  Slave2/1(OrionConnConfOut) -> DelaySwitch23/3(inMsg)
  Slave2/3(OrionKeepAliveOut) -> DelaySwitch21/3(inMsg)
  DelaySwitch24/1(outMsg) -> Master2/5(OrionConnRespIn)
  DelaySwitch25/1(outMsg) -> Master2/4(OrionAppDataIn)
  DelaySwitch23/1(outMsg) -> Master2/3(OrionConnConfIn)
  DelaySwitch21/1(outMsg) -> Master2/2(OrionKeepAliveIn)
  DelaySwitch22/1(outMsg) -> Slave2/4(OrionConnReqIn)
  DelaySwitch30/1(outMsg) -> Slave2/2(OrionAppDataIn)
  DelaySwitch29/1(outMsg) -> Slave2/3(OrionConnRespIn)
  DelaySwitch28/1(outMsg) -> Slave2/5(OrionConnConfIn)
  DelaySwitch27/1(outMsg) -> Slave2/1(OrionKeepAliveIn)
  Master2/6(connStatus) -> OverallState/5(conn5)
  Slave2/6(connStatus) -> OverallState/6(conn6)
  From Workspace44/1 -> DelaySwitch21/1(switch_array)
  From Workspace45/1 -> DelaySwitch21/2(delay_array)
  From Workspace59/1 -> DelaySwitch23/2(delay_array)
  From Workspace56/1 -> DelaySwitch23/1(switch_array)
  From Workspace60/1 -> DelaySwitch24/1(switch_array)
  From Workspace61/1 -> DelaySwitch24/2(delay_array)
  From Workspace63/1 -> DelaySwitch25/2(delay_array)
  From Workspace62/1 -> DelaySwitch25/1(switch_array)
  From Workspace64/1 -> DelaySwitch26/1(switch_array)
  From Workspace65/1 -> DelaySwitch26/2(delay_array)
  Slave2/5(OrionConnReqOut) -> DelaySwitch26/3(inMsg)
  DelaySwitch26/1(outMsg) -> Master2/6(OrionConnReqIn)
  From Workspace47/1 -> DelaySwitch27/2(delay_array)
  From Workspace46/1 -> DelaySwitch27/1(switch_array)
  Master2/1(OrionKeepAliveOut) -> DelaySwitch27/3(inMsg)
  From Workspace48/1 -> DelaySwitch28/1(switch_array)
  From Workspace49/1 -> DelaySwitch28/2(delay_array)
  From Workspace51/1 -> DelaySwitch29/2(delay_array)
  From Workspace50/1 -> DelaySwitch29/1(switch_array)
  Master2/2(OrionConnConfOut) -> DelaySwitch28/3(inMsg)
  Master2/3(OrionConnRespOut) -> DelaySwitch29/3(inMsg)
  From Workspace52/1 -> DelaySwitch30/1(switch_array)
  From Workspace53/1 -> DelaySwitch30/2(delay_array)
  From Workspace55/1 -> DelaySwitch22/2(delay_array)
  From Workspace54/1 -> DelaySwitch22/1(switch_array)
  Master2/4(OrionAppDataOut) -> DelaySwitch30/3(inMsg)
  Master2/5(OrionConnReqOut) -> DelaySwitch22/3(inMsg)
  From Workspace57/1 -> Slave2/6(delay_array)
  From Workspace58/1 -> Master2/1(delay_array)
  From Workspace80/1 -> Master3/1(delay_array)
  From Workspace79/1 -> Slave3/6(delay_array)
  Master3/5(OrionConnReqOut) -> DelaySwitch32/3(inMsg)
  Master3/4(OrionAppDataOut) -> DelaySwitch40/3(inMsg)
  From Workspace76/1 -> DelaySwitch32/1(switch_array)
  From Workspace77/1 -> DelaySwitch32/2(delay_array)
  From Workspace75/1 -> DelaySwitch40/2(delay_array)
  From Workspace74/1 -> DelaySwitch40/1(switch_array)
  Master3/3(OrionConnRespOut) -> DelaySwitch39/3(inMsg)
  Master3/2(OrionConnConfOut) -> DelaySwitch38/3(inMsg)
  From Workspace72/1 -> DelaySwitch39/1(switch_array)
  From Workspace73/1 -> DelaySwitch39/2(delay_array)
  From Workspace71/1 -> DelaySwitch38/2(delay_array)
  From Workspace70/1 -> DelaySwitch38/1(switch_array)
  Master3/1(OrionKeepAliveOut) -> DelaySwitch37/3(inMsg)
  From Workspace68/1 -> DelaySwitch37/1(switch_array)
  From Workspace69/1 -> DelaySwitch37/2(delay_array)
  DelaySwitch36/1(outMsg) -> Master3/6(OrionConnReqIn)
  Slave3/5(OrionConnReqOut) -> DelaySwitch36/3(inMsg)
  From Workspace87/1 -> DelaySwitch36/2(delay_array)
  From Workspace86/1 -> DelaySwitch36/1(switch_array)
  From Workspace84/1 -> DelaySwitch35/1(switch_array)
  From Workspace85/1 -> DelaySwitch35/2(delay_array)
  From Workspace83/1 -> DelaySwitch34/2(delay_array)
  From Workspace82/1 -> DelaySwitch34/1(switch_array)
  From Workspace78/1 -> DelaySwitch33/1(switch_array)
  From Workspace81/1 -> DelaySwitch33/2(delay_array)
  From Workspace67/1 -> DelaySwitch31/2(delay_array)
  From Workspace66/1 -> DelaySwitch31/1(switch_array)
  Slave3/6(connStatus) -> OverallState/8(conn8)
  Master3/6(connStatus) -> OverallState/7(conn7)
  DelaySwitch37/1(outMsg) -> Slave3/1(OrionKeepAliveIn)
  DelaySwitch38/1(outMsg) -> Slave3/5(OrionConnConfIn)
  DelaySwitch39/1(outMsg) -> Slave3/3(OrionConnRespIn)
  DelaySwitch40/1(outMsg) -> Slave3/2(OrionAppDataIn)
  DelaySwitch32/1(outMsg) -> Slave3/4(OrionConnReqIn)
  DelaySwitch31/1(outMsg) -> Master3/2(OrionKeepAliveIn)
  DelaySwitch33/1(outMsg) -> Master3/3(OrionConnConfIn)
  DelaySwitch35/1(outMsg) -> Master3/4(OrionAppDataIn)
  DelaySwitch34/1(outMsg) -> Master3/5(OrionConnRespIn)
  Slave3/3(OrionKeepAliveOut) -> DelaySwitch31/3(inMsg)
  Slave3/1(OrionConnConfOut) -> DelaySwitch33/3(inMsg)
  Slave3/2(OrionConnRespOut) -> DelaySwitch34/3(inMsg)
  Slave3/4(OrionAppDataOut) -> DelaySwitch35/3(inMsg)
  Slave7/4(OrionAppDataOut) -> DelaySwitch69/3(inMsg)
  Slave7/2(OrionConnRespOut) -> DelaySwitch68/3(inMsg)
  Slave7/1(OrionConnConfOut) -> DelaySwitch67/3(inMsg)
  Slave7/3(OrionKeepAliveOut) -> DelaySwitch65/3(inMsg)
  DelaySwitch68/1(outMsg) -> Master7/5(OrionConnRespIn)
  DelaySwitch69/1(outMsg) -> Master7/4(OrionAppDataIn)
  DelaySwitch67/1(outMsg) -> Master7/3(OrionConnConfIn)
  DelaySwitch65/1(outMsg) -> Master7/2(OrionKeepAliveIn)
  DelaySwitch66/1(outMsg) -> Slave7/4(OrionConnReqIn)
  DelaySwitch75/1(outMsg) -> Slave7/2(OrionAppDataIn)
  DelaySwitch73/1(outMsg) -> Slave7/3(OrionConnRespIn)
  DelaySwitch72/1(outMsg) -> Slave7/5(OrionConnConfIn)
  DelaySwitch71/1(outMsg) -> Slave7/1(OrionKeepAliveIn)
  Master7/6(connStatus) -> OverallState/16(conn16)
  Slave7/6(connStatus) -> OverallState/15(conn15)
  From Workspace151/1 -> DelaySwitch65/1(switch_array)
  From Workspace152/1 -> DelaySwitch65/2(delay_array)
  From Workspace168/1 -> DelaySwitch67/2(delay_array)
  From Workspace164/1 -> DelaySwitch67/1(switch_array)
  From Workspace169/1 -> DelaySwitch68/1(switch_array)
  From Workspace170/1 -> DelaySwitch68/2(delay_array)
  From Workspace172/1 -> DelaySwitch69/2(delay_array)
  From Workspace171/1 -> DelaySwitch69/1(switch_array)
  From Workspace173/1 -> DelaySwitch70/1(switch_array)
  From Workspace174/1 -> DelaySwitch70/2(delay_array)
  Slave7/5(OrionConnReqOut) -> DelaySwitch70/3(inMsg)
  DelaySwitch70/1(outMsg) -> Master7/6(OrionConnReqIn)
  From Workspace154/1 -> DelaySwitch71/2(delay_array)
  From Workspace153/1 -> DelaySwitch71/1(switch_array)
  Master7/1(OrionKeepAliveOut) -> DelaySwitch71/3(inMsg)
  From Workspace156/1 -> DelaySwitch72/1(switch_array)
  From Workspace157/1 -> DelaySwitch72/2(delay_array)
  From Workspace159/1 -> DelaySwitch73/2(delay_array)
  From Workspace158/1 -> DelaySwitch73/1(switch_array)
  Master7/2(OrionConnConfOut) -> DelaySwitch72/3(inMsg)
  Master7/3(OrionConnRespOut) -> DelaySwitch73/3(inMsg)
  From Workspace160/1 -> DelaySwitch75/1(switch_array)
  From Workspace161/1 -> DelaySwitch75/2(delay_array)
  From Workspace163/1 -> DelaySwitch66/2(delay_array)
  From Workspace162/1 -> DelaySwitch66/1(switch_array)
  Master7/4(OrionAppDataOut) -> DelaySwitch75/3(inMsg)
  Master7/5(OrionConnReqOut) -> DelaySwitch66/3(inMsg)
  From Workspace165/1 -> Slave7/6(delay_array)
  From Workspace167/1 -> Master7/1(delay_array)
  From Workspace142/1 -> Master6/1(delay_array)
  From Workspace141/1 -> Slave6/6(delay_array)
  Master6/5(OrionConnReqOut) -> DelaySwitch55/3(inMsg)
  Master6/4(OrionAppDataOut) -> DelaySwitch64/3(inMsg)
  From Workspace138/1 -> DelaySwitch55/1(switch_array)
  From Workspace139/1 -> DelaySwitch55/2(delay_array)
  From Workspace137/1 -> DelaySwitch64/2(delay_array)
  From Workspace136/1 -> DelaySwitch64/1(switch_array)
  Master6/3(OrionConnRespOut) -> DelaySwitch62/3(inMsg)
  Master6/2(OrionConnConfOut) -> DelaySwitch61/3(inMsg)
  From Workspace134/1 -> DelaySwitch62/1(switch_array)
  From Workspace135/1 -> DelaySwitch62/2(delay_array)
  From Workspace132/1 -> DelaySwitch61/2(delay_array)
  From Workspace131/1 -> DelaySwitch61/1(switch_array)
  Master6/1(OrionKeepAliveOut) -> DelaySwitch60/3(inMsg)
  From Workspace129/1 -> DelaySwitch60/1(switch_array)
  From Workspace130/1 -> DelaySwitch60/2(delay_array)
  DelaySwitch59/1(outMsg) -> Master6/6(OrionConnReqIn)
  Slave6/5(OrionConnReqOut) -> DelaySwitch59/3(inMsg)
  From Workspace150/1 -> DelaySwitch59/2(delay_array)
  From Workspace149/1 -> DelaySwitch59/1(switch_array)
  From Workspace147/1 -> DelaySwitch58/1(switch_array)
  From Workspace148/1 -> DelaySwitch58/2(delay_array)
  From Workspace146/1 -> DelaySwitch57/2(delay_array)
  From Workspace145/1 -> DelaySwitch57/1(switch_array)
  From Workspace140/1 -> DelaySwitch56/1(switch_array)
  From Workspace143/1 -> DelaySwitch56/2(delay_array)
  From Workspace128/1 -> DelaySwitch54/2(delay_array)
  From Workspace127/1 -> DelaySwitch54/1(switch_array)
  Slave6/6(connStatus) -> OverallState/14(conn14)
  Master6/6(connStatus) -> OverallState/13(conn13)
  DelaySwitch60/1(outMsg) -> Slave6/1(OrionKeepAliveIn)
  DelaySwitch61/1(outMsg) -> Slave6/5(OrionConnConfIn)
  DelaySwitch62/1(outMsg) -> Slave6/3(OrionConnRespIn)
  DelaySwitch64/1(outMsg) -> Slave6/2(OrionAppDataIn)
  DelaySwitch55/1(outMsg) -> Slave6/4(OrionConnReqIn)
  DelaySwitch54/1(outMsg) -> Master6/2(OrionKeepAliveIn)
  DelaySwitch56/1(outMsg) -> Master6/3(OrionConnConfIn)
  DelaySwitch58/1(outMsg) -> Master6/4(OrionAppDataIn)
  DelaySwitch57/1(outMsg) -> Master6/5(OrionConnRespIn)
  Slave6/3(OrionKeepAliveOut) -> DelaySwitch54/3(inMsg)
  Slave6/1(OrionConnConfOut) -> DelaySwitch56/3(inMsg)
  Slave6/2(OrionConnRespOut) -> DelaySwitch57/3(inMsg)
  Slave6/4(OrionAppDataOut) -> DelaySwitch58/3(inMsg)
  Slave5/4(OrionAppDataOut) -> DelaySwitch47/3(inMsg)
  Slave5/2(OrionConnRespOut) -> DelaySwitch46/3(inMsg)
  Slave5/1(OrionConnConfOut) -> DelaySwitch45/3(inMsg)
  Slave5/3(OrionKeepAliveOut) -> DelaySwitch43/3(inMsg)
  DelaySwitch46/1(outMsg) -> Master5/5(OrionConnRespIn)
  DelaySwitch47/1(outMsg) -> Master5/4(OrionAppDataIn)
  DelaySwitch45/1(outMsg) -> Master5/3(OrionConnConfIn)
  DelaySwitch43/1(outMsg) -> Master5/2(OrionKeepAliveIn)
  DelaySwitch44/1(outMsg) -> Slave5/4(OrionConnReqIn)
  DelaySwitch53/1(outMsg) -> Slave5/2(OrionAppDataIn)
  DelaySwitch51/1(outMsg) -> Slave5/3(OrionConnRespIn)
  DelaySwitch50/1(outMsg) -> Slave5/5(OrionConnConfIn)
  DelaySwitch49/1(outMsg) -> Slave5/1(OrionKeepAliveIn)
  Master5/6(connStatus) -> OverallState/11(conn11)
  Slave5/6(connStatus) -> OverallState/12(conn12)
  From Workspace103/1 -> DelaySwitch43/1(switch_array)
  From Workspace104/1 -> DelaySwitch43/2(delay_array)
  From Workspace119/1 -> DelaySwitch45/2(delay_array)
  From Workspace116/1 -> DelaySwitch45/1(switch_array)
  From Workspace120/1 -> DelaySwitch46/1(switch_array)
  From Workspace121/1 -> DelaySwitch46/2(delay_array)
  From Workspace124/1 -> DelaySwitch47/2(delay_array)
  From Workspace123/1 -> DelaySwitch47/1(switch_array)
  From Workspace125/1 -> DelaySwitch48/1(switch_array)
  From Workspace126/1 -> DelaySwitch48/2(delay_array)
  Slave5/5(OrionConnReqOut) -> DelaySwitch48/3(inMsg)
  DelaySwitch48/1(outMsg) -> Master5/6(OrionConnReqIn)
  From Workspace106/1 -> DelaySwitch49/2(delay_array)
  From Workspace105/1 -> DelaySwitch49/1(switch_array)
  Master5/1(OrionKeepAliveOut) -> DelaySwitch49/3(inMsg)
  From Workspace107/1 -> DelaySwitch50/1(switch_array)
  From Workspace108/1 -> DelaySwitch50/2(delay_array)
  From Workspace110/1 -> DelaySwitch51/2(delay_array)
  From Workspace109/1 -> DelaySwitch51/1(switch_array)
  Master5/2(OrionConnConfOut) -> DelaySwitch50/3(inMsg)
  Master5/3(OrionConnRespOut) -> DelaySwitch51/3(inMsg)
  From Workspace112/1 -> DelaySwitch53/1(switch_array)
  From Workspace113/1 -> DelaySwitch53/2(delay_array)
  From Workspace115/1 -> DelaySwitch44/2(delay_array)
  From Workspace114/1 -> DelaySwitch44/1(switch_array)
  Master5/4(OrionAppDataOut) -> DelaySwitch53/3(inMsg)
  Master5/5(OrionConnReqOut) -> DelaySwitch44/3(inMsg)
  From Workspace117/1 -> Slave5/6(delay_array)
  From Workspace118/1 -> Master5/1(delay_array)
  From Workspace102/1 -> Master4/1(delay_array)
  From Workspace101/1 -> Slave4/6(delay_array)
  Master4/5(OrionConnReqOut) -> DelaySwitch42/3(inMsg)
  Master4/4(OrionAppDataOut) -> DelaySwitch80/3(inMsg)
  From Workspace98/1 -> DelaySwitch42/1(switch_array)
  From Workspace99/1 -> DelaySwitch42/2(delay_array)
  From Workspace97/1 -> DelaySwitch80/2(delay_array)
  From Workspace96/1 -> DelaySwitch80/1(switch_array)
  Master4/3(OrionConnRespOut) -> DelaySwitch79/3(inMsg)
  Master4/2(OrionConnConfOut) -> DelaySwitch78/3(inMsg)
  From Workspace94/1 -> DelaySwitch79/1(switch_array)
  From Workspace95/1 -> DelaySwitch79/2(delay_array)
  From Workspace93/1 -> DelaySwitch78/2(delay_array)
  From Workspace92/1 -> DelaySwitch78/1(switch_array)
  Master4/1(OrionKeepAliveOut) -> DelaySwitch77/3(inMsg)
  From Workspace90/1 -> DelaySwitch77/1(switch_array)
  From Workspace91/1 -> DelaySwitch77/2(delay_array)
  DelaySwitch76/1(outMsg) -> Master4/6(OrionConnReqIn)
  Slave4/5(OrionConnReqOut) -> DelaySwitch76/3(inMsg)
  From Workspace175/1 -> DelaySwitch76/2(delay_array)
  From Workspace166/1 -> DelaySwitch76/1(switch_array)
  From Workspace144/1 -> DelaySwitch74/1(switch_array)
  From Workspace155/1 -> DelaySwitch74/2(delay_array)
  From Workspace133/1 -> DelaySwitch63/2(delay_array)
  From Workspace122/1 -> DelaySwitch63/1(switch_array)
  From Workspace100/1 -> DelaySwitch52/1(switch_array)
  From Workspace111/1 -> DelaySwitch52/2(delay_array)
  From Workspace89/1 -> DelaySwitch41/2(delay_array)
  From Workspace88/1 -> DelaySwitch41/1(switch_array)
  Slave4/6(connStatus) -> OverallState/10(conn10)
  Master4/6(connStatus) -> OverallState/9(conn9)
  DelaySwitch77/1(outMsg) -> Slave4/1(OrionKeepAliveIn)
  DelaySwitch78/1(outMsg) -> Slave4/5(OrionConnConfIn)
  DelaySwitch79/1(outMsg) -> Slave4/3(OrionConnRespIn)
  DelaySwitch80/1(outMsg) -> Slave4/2(OrionAppDataIn)
  DelaySwitch42/1(outMsg) -> Slave4/4(OrionConnReqIn)
  DelaySwitch41/1(outMsg) -> Master4/2(OrionKeepAliveIn)
  DelaySwitch52/1(outMsg) -> Master4/3(OrionConnConfIn)
  DelaySwitch74/1(outMsg) -> Master4/4(OrionAppDataIn)
  DelaySwitch63/1(outMsg) -> Master4/5(OrionConnRespIn)
  Slave4/3(OrionKeepAliveOut) -> DelaySwitch41/3(inMsg)
  Slave4/1(OrionConnConfOut) -> DelaySwitch52/3(inMsg)
  Slave4/2(OrionConnRespOut) -> DelaySwitch63/3(inMsg)
  Slave4/4(OrionAppDataOut) -> DelaySwitch74/3(inMsg)
